simulink model "Approach"  (R2017a)
settings: Solver=VariableStepAuto  StartTime=0.0  StopTime=500  RelTol=1e-3
libraries: cstblocks x3
settings Model: Creator=user  LastModifiedBy=user

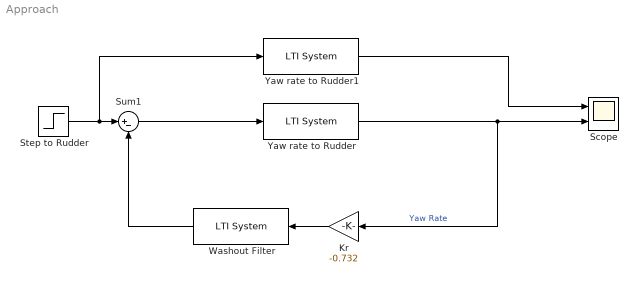
== system Approach ==
  Kr : Gain  Gain=-0.732
  Scope : Scope  NumInputPorts=2
  Step to Rudder : Step  SampleTime=0
  Sum1 : Sum  Inputs=|+-
  Washout Filter : cstblocks/LTI System  sys=Filter  IC=[]
  Yaw rate to Rudder : cstblocks/LTI System  sys=Sys23  IC=[]
  Yaw rate to Rudder1 : cstblocks/LTI System  sys=Sys23  IC=[]
  wires:
  Yaw rate to Rudder1/1 -> Scope/1
  Step to Rudder/1 -> Yaw rate to Rudder1/1, Sum1/1
  Yaw rate to Rudder/1 -> Kr/1, Scope/2  "Yaw Rate"
  Washout Filter/1 -> Sum1/2
  Kr/1 -> Washout Filter/1
  Sum1/1 -> Yaw rate to Rudder/1
